simulink model "r4_pfb_fir"  (Simulink 7.0)
settings: Solver=FixedStepDiscrete  SolverMode=SingleTasking  StartTime=0.0  StopTime=10.0  RelTol=1e-3
undefined symbols (not defined in the file): pfb_coefs
libraries: xbsIndex_r4 x385, xps_library x1
(part 15 of 27)

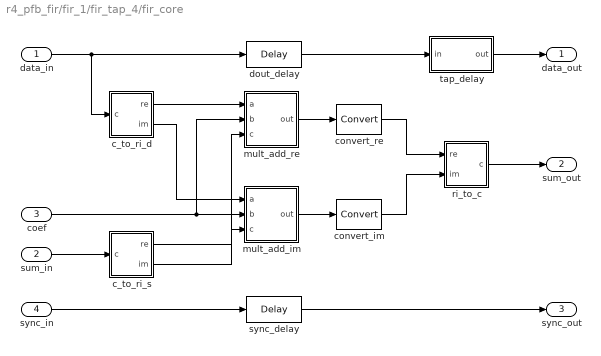
== system r4_pfb_fir/fir_1/fir_tap_4/fir_core ==
  data_in : Inport  OutDataType=sfix(16)  OutScaling=2^0
  sum_in : Inport  Port=2  OutDataType=sfix(16)  OutScaling=2^0
  coef : Inport  Port=3  OutDataType=sfix(16)  OutScaling=2^0
  sync_in : Inport  Port=4  OutDataType=sfix(16)  OutScaling=2^0
  c_to_ri_d : Subsystem  mask(Complex to Real-Imag){n_bits=8, bin_pt=7}
      mask prompts: n_bits "Bit Width"; bin_pt "Binary Point"
      mask help: Outputs real and imaginary components of a complex input.
      settings: AttributesFormatString=8_7 r/i
      mask Help:
      | <pre>
      | Description::
      | 
      | Outputs real and imaginary components of a complex input.
      | Useful for simplifying interconnects.
      | See also: Real-Imag to Complex (ri_to_c)
      | 
      | Mask Parameters::
      | 
      | Bit Width (n_bits): Specifies the width of the real/imaginary components.
      | Assumed equal for both components.
      | 
      | Binary Point (bin_pt): Specifies the binary point location in the real/imaginary components.
      | Assumed equal for both components.
      | </pre>
  c_to_ri_s : Subsystem  mask(Complex to Real-Imag){n_bits=17, bin_pt=15}
      mask prompts: n_bits "Bit Width"; bin_pt "Binary Point"
      mask help: Outputs real and imaginary components of a complex input.
      settings: AttributesFormatString=17_15 r/i
      mask Help:
      | <pre>
      | Description::
      | 
      | Outputs real and imaginary components of a complex input.
      | Useful for simplifying interconnects.
      | See also: Real-Imag to Complex (ri_to_c)
      | 
      | Mask Parameters::
      | 
      | Bit Width (n_bits): Specifies the width of the real/imaginary components.
      | Assumed equal for both components.
      | 
      | Binary Point (bin_pt): Specifies the binary point location in the real/imaginary components.
      | Assumed equal for both components.
      | </pre>
  convert_im : xbsIndex_r4/Convert  arith_type="Signed  (2's comp)"  n_bits=17  bin_pt=15  quantization=Truncate  overflow=Wrap  latency=0  dbl_ovrd=off  pipeline=on  block_type=convert
      settings: xl_area=[0, 0, 0, 0, 0, 0, 0]  block_version=10.1.3
  convert_re : xbsIndex_r4/Convert  arith_type="Signed  (2's comp)"  n_bits=17  bin_pt=15  quantization=Truncate  overflow=Wrap  latency=0  dbl_ovrd=off  pipeline=on  block_type=convert
      settings: xl_area=[0, 0, 0, 0, 0, 0, 0]  block_version=10.1.3
  dout_delay : xbsIndex_r4/Delay  en=off  latency=4  dbl_ovrd=off  reg_retiming=off  block_type=delay
      settings: xl_area=[0, 0, 0, 0, 0, 0, 0]
  mult_add_im : Subsystem  mask(Multiply Add Block){mult_latency=3, add_latency=1, add_bypass=off}
      mask prompts: mult_latency "Multiplier Latency"; add_latency "Adder Latency"; add_bypass "Bypass Adder"
      mask help: A full precision multiply-add block. Produces a*b+c at its ab_c output. The add operation can be optionally bypassed.
      settings: AttributesFormatString=|
      | out = a*b+c
      | latency = 4
      mask Help:
      | <pre>
      | Description::
      | 
      | This full precision multiply-add block produces a*b+c at its ab_c output.
      | The add operation can be optionally bypassed.
      | 
      | Latency is one multiplier latency plus one adder latency (if not bypassing adder).
      | 
      | Mask Parameters::
      | 
      | Multiplier Latency (mult_latency): Latency to use for the underlying real multipliers.
      | 
      | Adder Latency (add_latency): Latency to use for the underlying real adders.
      | 
      | Bypass Adder (add_bypass): Check this checkbox to bypass the adder.
      | </pre>
  mult_add_re : Subsystem  mask(Multiply Add Block){mult_latency=3, add_latency=1, add_bypass=off}
      mask prompts: mult_latency "Multiplier Latency"; add_latency "Adder Latency"; add_bypass "Bypass Adder"
      mask help: A full precision multiply-add block. Produces a*b+c at its ab_c output. The add operation can be optionally bypassed.
      settings: AttributesFormatString=|
      | out = a*b+c
      | latency = 4
      mask Help:
      | <pre>
      | Description::
      | 
      | This full precision multiply-add block produces a*b+c at its ab_c output.
      | The add operation can be optionally bypassed.
      | 
      | Latency is one multiplier latency plus one adder latency (if not bypassing adder).
      | 
      | Mask Parameters::
      | 
      | Multiplier Latency (mult_latency): Latency to use for the underlying real multipliers.
      | 
      | Adder Latency (add_latency): Latency to use for the underlying real adders.
      | 
      | Bypass Adder (add_bypass): Check this checkbox to bypass the adder.
      | </pre>
  ri_to_c : Subsystem  mask(Real-Imag to Complex){}
      mask help: Concatenates real and imaginary inputs into a complex output.
      mask init:
      | ri_to_c_init(gcb);
      mask Help:
      | <pre>
      | Description::
      | 
      | Concatenates a real and imaginary input into a complex output.
      | Useful for simplifying interconnects.
      | See also: Complex to Real-Imag (c_to_ri)
      | 
      | Mask Parameters::
      | 
      | (N/A)
      | </pre>
  sync_delay : xbsIndex_r4/Delay  en=off  latency=4  dbl_ovrd=off  reg_retiming=off  block_type=delay
      settings: xl_area=[0, 0, 0, 0, 0, 0, 0]
  tap_delay : Subsystem  mask(BRAM Delay){delay_depth=1024, buffer_latency=}
      mask prompts: delay_depth "Delay Depth"; buffer_latency "Buffer Latency"
      mask help: A delay block that uses BRAM for its storage.
      settings: AttributesFormatString=bram depth = 1024
      mask Help:
      | <pre>
      | Description::
      | 
      | A delay block that uses BRAM for its storage.
      | 
      | Mask Parameters::
      | 
      | Delay Depth (delay_depth): The length of the delay.
      | 
      | Buffer Latency (buffer_latency): The latency of the underlying storage.
      | 
      | Buffer Latency defaults to 1 and cannot be changed via the block's dialog box.
      | Future versions may enable the setting of that parameter from the dialog.
      | </pre>
  data_out : Outport  OutDataType=sfix(16)  OutScaling=2^0
  sum_out : Outport  Port=2  OutDataType=sfix(16)  OutScaling=2^0
  sync_out : Outport  Port=3  OutDataType=sfix(16)  OutScaling=2^0
  wires:
  convert_im/1 -> ri_to_c/2(im)
  convert_re/1 -> ri_to_c/1(re)
  tap_delay/1(out) -> data_out/1
  mult_add_im/1(out) -> convert_im/1
  mult_add_re/1(out) -> convert_re/1
  c_to_ri_s/2(im) -> mult_add_im/3(c)
  c_to_ri_s/1(re) -> mult_add_re/3(c)
  sum_in/1 -> c_to_ri_s/1(c)
  coef/1 -> mult_add_re/2(b), mult_add_im/2(b)
  c_to_ri_d/2(im) -> mult_add_im/1(a)
  c_to_ri_d/1(re) -> mult_add_re/1(a)
  data_in/1 -> c_to_ri_d/1(c), dout_delay/1
  dout_delay/1 -> tap_delay/1(in)
  ri_to_c/1(c) -> sum_out/1
  sync_delay/1 -> sync_out/1
  sync_in/1 -> sync_delay/1

== system r4_pfb_fir/fir_1/fir_tap_5/fir_coef ==
  data_in : Inport  OutDataType=sfix(16)  OutScaling=2^0
  sum_in : Inport  Port=2  OutDataType=sfix(16)  OutScaling=2^0
  sync_in : Inport  Port=3  OutDataType=sfix(16)  OutScaling=2^0
  c_gen : Subsystem  mask(Coefficient Generator){coefs=[-7.57186305694141e-005;-0.000227564945670749;-0.000379956430889435;-0.000532892796251757;-0.000686373742881339;-0.000840398962979647;-0.000994968139806186;-0.00115008094765919;-0.00130573705185642;-0.00146193610871559;-0.00161867776553536;-0.00177596166057639;-0.00193378742304204;-0.0020921546730598;-0.0022510630216622;-0.00241051207076825;-0.00257050141316491;-0.00273103063248833;-0.00289209930320557;-0.00305370699059638;-0.00321585325073467;-0.00337853763047057;-0.00354175966741245;-0.00370551888990871;-0.00386981481703025;-0.00403464695855241;-0.00420001481493748;-0.00436591787731722;-0.0045323556274752;-0.00469932753782952;-0.00486683307141569;-0.00503487168186923;-0.00520344281340873;-0.00537254590081901;-0.00554218036943399;-0.00571234563512023;-0.00588304110426002;-0.00605426617373492;-0.00622602023090949;-0.00639830265361464;-0.00657111281013151;-0.00674445005917552;-0.00691831374988003;-0.00709270322178053;-0.00726761780479901;-0.00744305681922785;-0.00761901957571464;-0.00779550537524631;-0.0079725135091339;-0.00815004325899737;-0.00832809389675017;-0.0085066646845843;-0.00868575487495546;-0.00886536371056795;-0.00904549042435999;-0.00922613423948933;-0.00940729436931827;-0.0095889700173997;-0.00977116037746245;-0.00995386463339719;-0.0101370819592425;-0.0103208115191707;-0.010505052467474;-0.0106898039485508;-0.0108750650968923;-0.0110608350370682;-0.0112471128837145;-0.011433897741519;-0.0116211887052088;-0.0118089848595372;-0.0119972852792704;-0.0121860890291751;-0.0123753951640054;-0.0125652027284904;-0.0127555107573218;-0.0129463182751411;-0.013137624296528;-0.0133294278259877;-0.0135217278579391;-0.013714523376703;-0.0139078133564902;-0.0141015967613896;-0.0142958725453573;-0.0144906396522044;-0.0146858970155864;-0.0148816435589916;-0.01507787819573;-0.0152745998289226;-0.0154718073514906;-0.0156694996461444;-0.0158676755853733;-0.016066334031435;-0.016265473836345;-0.0164650938418669;-0.016665192879502;-0.0168657697704791;-0.0170668233257453;-0.0172683523459559;-0.0174703556214645;-0.0176728319323143;-0.0178757800482282;-0.0180791987285998;-0.0182830867224842;-0.018487442768589;-0.0186922655952659;-0.0188975539205014;-0.0191033064519087;-0.019309521886719;-0.0195161989117731;-0.0197233362035136;-0.0199309324279764;-0.0201389862407831;-0.020347496287133;-0.0205564612017955;-0.0207658796091025;-0.0209757501229411;-0.0211860713467461;-0.0213968418734932;-0.0216080602856917;-0.0218197251553776;-0.022031835044107;-0.0222443885029495;-0.0224573840724814;-0.0226708202827797;-0.0228846956534157;-0.0230990086934489;-0.0233137579014212;-0.0235289417653507;-0.0237445587627263;-0.0239606073605024;-0.0241770860150929;-0.024393993172366;-0.0246113272676396;-0.0248290867256759;-0.025047269960676;-0.0252658753762764;-0.0254849013655432;-0.0257043463109681;-0.0259242085844644;-0.026144486547362;-0.0263651785504042;-0.026586282933743;-0.026807798026936;-0.0270297221489423;-0.0272520536081191;-0.0274747907022183;-0.0276979317183836;-0.0279214749331467;-0.0281454186124251;-0.0283697610115189;-0.0285945003751079;-0.0288196349372498;-0.029045162921377;-0.0292710825402948;-0.0294973919961793;-0.0297240894805752;-0.0299511731743939;-0.0301786412479123;-0.0304064918607708;-0.0306347231619722;-0.03086333328988;-0.0310923203722177;-0.0313216825260677;-0.0315514178578704;-0.0317815244634236;-0.0320120004278819;-0.0322428438257562;-0.0324740527209136;-0.0327056251665774;-0.0329375592053265;-0.0331698528690966;-0.0334025041791795;-0.0336355111462241;-0.0338688717702371;-0.0341025840405833;-0.0343366459359869;-0.0345710554245323;-0.0348058104636656;-0.0350409090001953;-0.0352763489702948;-0.035512128299503;-0.0357482449027266;-0.0359846966842419;-0.036221481537697;-0.036458597346114;-0.0366960419818909;-0.0369338133068049;-0.0371719091720144;-0.0374103274180622;-0.037649065874878;-0.0378881223617824;-0.038127494687489;-0.0383671806501086;-0.0386071780371525;-0.0388474846255361;-0.0390880981815831;-0.039329016461029;-0.0395702372090256 ...(+16053 chars)], n_bits=9, bin_pt=8, log2_cpc=0, use_bram=on}
      mask prompts: coefs "Coefficients"; n_bits "Number of Bits"; bin_pt "Binary Point"; log2_cpc "Log2 Cycles per Coefficient"; use_bram "Use BRAM"
      mask help: A coefficient generator.
      settings: AttributesFormatString=|
      | 1024 coefs in bram
      | 9_8 out/1
      mask Help:
      | <pre>
      | Description::
      | 
      | A coefficient generator.
      | 
      | Mask Parameters::
      | 
      | Coefficiants (coefs): The coefficients to output.  These should be specified as doubles.
      | They will be rounded/saturated according to the specified number of bits (n_bits)
      | and binary point (bin_pt).
      | 
      | Number of Coefficient Bits (n_bits): The number of bits used for the fixed point binary
      | representation of the coefficients.
      | 
      | Coefficient Binary Point (bin_pt): The binary point of the fixed point binary representation
      | of the coefficients.
      | 
      | Log2 Cycles per Coefficient (log2_cpc): The log2 value of the number of cycles per coefficient.
      | Must be a non-negative integer (i.e. cycles per coefficient must be a power of 2).
      | 
      | Use BRAM (use_bram): Check this checkbox to store coefficients in BRAM.
      | If unchecked, the coefficients will be sored in distributed memory (i.e. slices).
      | </pre>
  data_delay : xbsIndex_r4/Delay  en=off  latency=1  dbl_ovrd=off  reg_retiming=off  block_type=delay
      settings: xl_area=[0, 0, 0, 0, 0, 0, 0]
  sum_delay : xbsIndex_r4/Delay  en=off  latency=1  dbl_ovrd=off  reg_retiming=off  block_type=delay
      settings: xl_area=[0, 0, 0, 0, 0, 0, 0]
  sync_delay : xbsIndex_r4/Delay  en=off  latency=1  dbl_ovrd=off  reg_retiming=off  block_type=delay
      settings: xl_area=[0, 0, 0, 0, 0, 0, 0]
  data_out : Outport  OutDataType=sfix(16)  OutScaling=2^0
  sum_out : Outport  Port=2  OutDataType=sfix(16)  OutScaling=2^0
  coef : Outport  Port=3  OutDataType=sfix(16)  OutScaling=2^0
  sync_out : Outport  Port=4  OutDataType=sfix(16)  OutScaling=2^0
  wires:
  c_gen/1(coef_out) -> coef/1
  sum_delay/1 -> sum_out/1
  sum_in/1 -> sum_delay/1
  sync_in/1 -> c_gen/1(sync_in), sync_delay/1
  sync_delay/1 -> sync_out/1
  data_delay/1 -> data_out/1
  data_in/1 -> data_delay/1

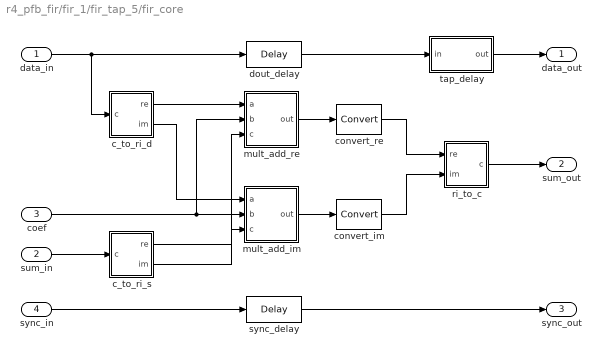
== system r4_pfb_fir/fir_1/fir_tap_5/fir_core ==
  data_in : Inport  OutDataType=sfix(16)  OutScaling=2^0
  sum_in : Inport  Port=2  OutDataType=sfix(16)  OutScaling=2^0
  coef : Inport  Port=3  OutDataType=sfix(16)  OutScaling=2^0
  sync_in : Inport  Port=4  OutDataType=sfix(16)  OutScaling=2^0
  c_to_ri_d : Subsystem  mask(Complex to Real-Imag){n_bits=8, bin_pt=7}
      mask prompts: n_bits "Bit Width"; bin_pt "Binary Point"
      mask help: Outputs real and imaginary components of a complex input.
      settings: AttributesFormatString=8_7 r/i
      mask Help:
      | <pre>
      | Description::
      | 
      | Outputs real and imaginary components of a complex input.
      | Useful for simplifying interconnects.
      | See also: Real-Imag to Complex (ri_to_c)
      | 
      | Mask Parameters::
      | 
      | Bit Width (n_bits): Specifies the width of the real/imaginary components.
      | Assumed equal for both components.
      | 
      | Binary Point (bin_pt): Specifies the binary point location in the real/imaginary components.
      | Assumed equal for both components.
      | </pre>
  c_to_ri_s : Subsystem  mask(Complex to Real-Imag){n_bits=17, bin_pt=15}
      mask prompts: n_bits "Bit Width"; bin_pt "Binary Point"
      mask help: Outputs real and imaginary components of a complex input.
      settings: AttributesFormatString=17_15 r/i
      mask Help:
      | <pre>
      | Description::
      | 
      | Outputs real and imaginary components of a complex input.
      | Useful for simplifying interconnects.
      | See also: Real-Imag to Complex (ri_to_c)
      | 
      | Mask Parameters::
      | 
      | Bit Width (n_bits): Specifies the width of the real/imaginary components.
      | Assumed equal for both components.
      | 
      | Binary Point (bin_pt): Specifies the binary point location in the real/imaginary components.
      | Assumed equal for both components.
      | </pre>
  convert_im : xbsIndex_r4/Convert  arith_type="Signed  (2's comp)"  n_bits=17  bin_pt=15  quantization=Truncate  overflow=Wrap  latency=0  dbl_ovrd=off  pipeline=on  block_type=convert
      settings: xl_area=[0, 0, 0, 0, 0, 0, 0]  block_version=10.1.3
  convert_re : xbsIndex_r4/Convert  arith_type="Signed  (2's comp)"  n_bits=17  bin_pt=15  quantization=Truncate  overflow=Wrap  latency=0  dbl_ovrd=off  pipeline=on  block_type=convert
      settings: xl_area=[0, 0, 0, 0, 0, 0, 0]  block_version=10.1.3
  dout_delay : xbsIndex_r4/Delay  en=off  latency=4  dbl_ovrd=off  reg_retiming=off  block_type=delay
      settings: xl_area=[0, 0, 0, 0, 0, 0, 0]
  mult_add_im : Subsystem  mask(Multiply Add Block){mult_latency=3, add_latency=1, add_bypass=off}
      mask prompts: mult_latency "Multiplier Latency"; add_latency "Adder Latency"; add_bypass "Bypass Adder"
      mask help: A full precision multiply-add block. Produces a*b+c at its ab_c output. The add operation can be optionally bypassed.
      settings: AttributesFormatString=|
      | out = a*b+c
      | latency = 4
      mask Help:
      | <pre>
      | Description::
      | 
      | This full precision multiply-add block produces a*b+c at its ab_c output.
      | The add operation can be optionally bypassed.
      | 
      | Latency is one multiplier latency plus one adder latency (if not bypassing adder).
      | 
      | Mask Parameters::
      | 
      | Multiplier Latency (mult_latency): Latency to use for the underlying real multipliers.
      | 
      | Adder Latency (add_latency): Latency to use for the underlying real adders.
      | 
      | Bypass Adder (add_bypass): Check this checkbox to bypass the adder.
      | </pre>
  mult_add_re : Subsystem  mask(Multiply Add Block){mult_latency=3, add_latency=1, add_bypass=off}
      mask prompts: mult_latency "Multiplier Latency"; add_latency "Adder Latency"; add_bypass "Bypass Adder"
      mask help: A full precision multiply-add block. Produces a*b+c at its ab_c output. The add operation can be optionally bypassed.
      settings: AttributesFormatString=|
      | out = a*b+c
      | latency = 4
      mask Help:
      | <pre>
      | Description::
      | 
      | This full precision multiply-add block produces a*b+c at its ab_c output.
      | The add operation can be optionally bypassed.
      | 
      | Latency is one multiplier latency plus one adder latency (if not bypassing adder).
      | 
      | Mask Parameters::
      | 
      | Multiplier Latency (mult_latency): Latency to use for the underlying real multipliers.
      | 
      | Adder Latency (add_latency): Latency to use for the underlying real adders.
      | 
      | Bypass Adder (add_bypass): Check this checkbox to bypass the adder.
      | </pre>
  ri_to_c : Subsystem  mask(Real-Imag to Complex){}
      mask help: Concatenates real and imaginary inputs into a complex output.
      mask init:
      | ri_to_c_init(gcb);
      mask Help:
      | <pre>
      | Description::
      | 
      | Concatenates a real and imaginary input into a complex output.
      | Useful for simplifying interconnects.
      | See also: Complex to Real-Imag (c_to_ri)
      | 
      | Mask Parameters::
      | 
      | (N/A)
      | </pre>
  sync_delay : xbsIndex_r4/Delay  en=off  latency=4  dbl_ovrd=off  reg_retiming=off  block_type=delay
      settings: xl_area=[0, 0, 0, 0, 0, 0, 0]
  tap_delay : Subsystem  mask(BRAM Delay){delay_depth=1024, buffer_latency=}
      mask prompts: delay_depth "Delay Depth"; buffer_latency "Buffer Latency"
      mask help: A delay block that uses BRAM for its storage.
      settings: AttributesFormatString=bram depth = 1024
      mask Help:
      | <pre>
      | Description::
      | 
      | A delay block that uses BRAM for its storage.
      | 
      | Mask Parameters::
      | 
      | Delay Depth (delay_depth): The length of the delay.
      | 
      | Buffer Latency (buffer_latency): The latency of the underlying storage.
      | 
      | Buffer Latency defaults to 1 and cannot be changed via the block's dialog box.
      | Future versions may enable the setting of that parameter from the dialog.
      | </pre>
  data_out : Outport  OutDataType=sfix(16)  OutScaling=2^0
  sum_out : Outport  Port=2  OutDataType=sfix(16)  OutScaling=2^0
  sync_out : Outport  Port=3  OutDataType=sfix(16)  OutScaling=2^0
  wires:
  convert_im/1 -> ri_to_c/2(im)
  convert_re/1 -> ri_to_c/1(re)
  tap_delay/1(out) -> data_out/1
  mult_add_im/1(out) -> convert_im/1
  mult_add_re/1(out) -> convert_re/1
  c_to_ri_s/2(im) -> mult_add_im/3(c)
  c_to_ri_s/1(re) -> mult_add_re/3(c)
  sum_in/1 -> c_to_ri_s/1(c)
  coef/1 -> mult_add_re/2(b), mult_add_im/2(b)
  c_to_ri_d/2(im) -> mult_add_im/1(a)
  c_to_ri_d/1(re) -> mult_add_re/1(a)
  data_in/1 -> c_to_ri_d/1(c), dout_delay/1
  dout_delay/1 -> tap_delay/1(in)
  ri_to_c/1(c) -> sum_out/1
  sync_delay/1 -> sync_out/1
  sync_in/1 -> sync_delay/1
